simulink model "L_21_05_11_reti_anticipatrici_schema"  (R2021b)
settings: Solver=VariableStepAuto  StartTime=0.0  StopTime=10  RelTol=1e-3
values from neighbouring files (symbols this model uses):
  Kr = 1    [L_11_05_21_reti_anticipatrici.m]    (also in L_11_05_21_reti_anticipatrici_2.m; L_12_05_21_Esercizio_progetto_di_un_controllore.m; L_12_05_21_effetti_sul_comando.m; L_12_05_21_reti_integro-derivative.m)
libraries: cstblocks x2, simulink x1
settings Model: Creator=francescafornasier  LastModifiedBy=francescafornasier

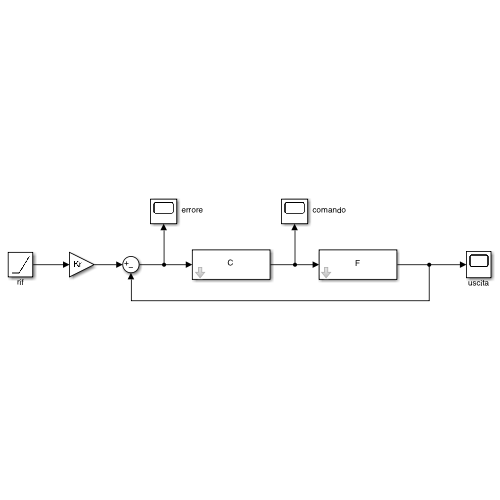
[thumbnail: Simulink's stored preview of the top-level diagram]
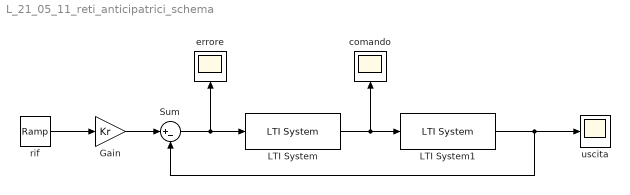
== system L_21_05_11_reti_anticipatrici_schema ==
  Gain : Gain  Gain=Kr
  LTI System : cstblocks/LTI System  sys=C  IC=[]
  LTI System1 : cstblocks/LTI System  sys=F  IC=[]
  Sum : Sum  Inputs=|+-
  comando : Scope
  errore : Scope
  rif : simulink/Sources/Ramp  slope=1  start=0  InitialOutput=0
  uscita : Scope
  wires:
  rif/1 -> Gain/1
  Gain/1 -> Sum/1
  Sum/1 -> LTI System/1, errore/1
  LTI System1/1 -> Sum/2, uscita/1
  LTI System/1 -> LTI System1/1, comando/1
